simulink model "air_conditioner"  (R2014a)
settings: Solver=ode45  StartTime=0.0  StopTime=inf  RelTol=1e-3
settings Model: Creator=feisele  LastModifiedBy=feisele

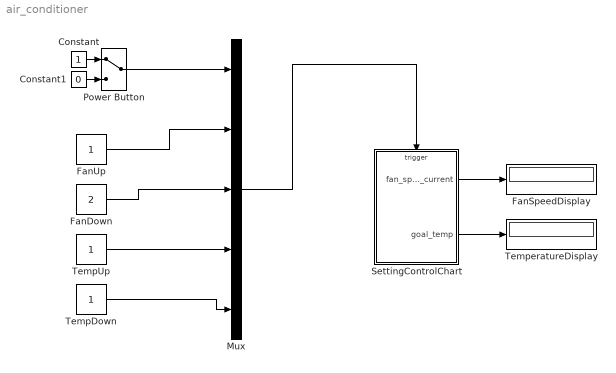
== system air_conditioner ==
  Constant : Constant
  Constant1 : Constant  Value=0
  FanDown : Constant  Value=2
  FanSpeedDisplay : Display
  FanUp : Constant
  Mux : Mux  Inputs=5
  Power Button : ManualSwitch
  SettingControlChart : Stateflow chart  TreatAsAtomicUnit=on
  TempDown : Constant
  TempUp : Constant
  TemperatureDisplay : Display
  wires:
  Power Button/1 -> Mux/1
  Constant/1 -> Power Button/1
  Constant1/1 -> Power Button/2
  SettingControlChart/1(fan_speed_current) -> FanSpeedDisplay/1
  SettingControlChart/2(goal_temp) -> TemperatureDisplay/1
  FanUp/1 -> Mux/2
  Mux/1 -> SettingControlChart/Trigger
  FanDown/1 -> Mux/3
  TempUp/1 -> Mux/4
  TempDown/1 -> Mux/5

== stateflow chart air_conditioner/SettingControlChart ==
  settings: executeAtInitialization=1
  state Power_on
    state Fan_setting [parallel]
      settings: executionOrder=2
      state Fan
      Fan -> Fan [order 1] : fan_up [fan_speed_current < MAXF]
          | { fan_speed_current = fan_speed_current + 1;
          | manual_on }
      (default) -> Fan
      Fan -> Fan [order 2] : fan_down [MINF < fan_speed_current]
          | { fan_speed_current = fan_speed_current - 1;
          | manual_on }
    state Mode_setting [parallel]
      settings: executionOrder=3
      state ManualMode
      state Computed_mode
        state Auto_mode
        state Turboo_mode
        (default) -> Auto_mode
      Computed_mode -> ManualMode : manual_on
          | { fan_speed_current = manual_fan;;
          | goal_temp = manual_temp }
      Mode_setting -> Auto_mode [order 2] : auto_on
          | { fan_speed_curren = auto_fan }
      Mode_setting -> Turboo_mode [order 1] : turbo_on
          | { fan_speed_current = MAXF;
          | goal_temp = MAXT };
    state Temperature_setting [parallel]
      settings: executionOrder=1
      state Temp
      Temp -> Temp [order 1] : temp_up [goal_temp < MAXT]
          | { goal_temp = goal_temp + 1 }
      (default) -> Temp
      Temp -> Temp [order 2] : temp_down [MINT < goal_temp]
          | { goal_temp = goal_temp -1 }
  state Power_off
  Power_off -> Power_on : { fan_speed_current = 1;
      | goal_temp = 2  }
  (default) -> Power_off
  Power_on -> Power_off : power_press
  data: MAXF constant uint8; MINF constant uint8; MINT constant uint8; MAXT constant uint8; fan_speed_current output; goal_temp output
  events: power_press input EITHER_EDGE_EVENT; manual_on local FUNCTION_CALL_EVENT; fan_up input RISING_EDGE_EVENT; fan_down input RISING_EDGE_EVENT; temp_up input RISING_EDGE_EVENT; temp_down input RISING_EDGE_EVENT
